simulink model "test_individual_beam_backup"  (R2013a)
settings: Solver=ode14x  StartTime=0.0  StopTime=3  FixedStep=1e-4  RelTol=1e-3
values from neighbouring files (symbols this model uses):
  A = [0 1 0 0 0 0;-2 0 2 0 0 0;0 0 0 1 0 0;2 0 -4 -3 2 3;0 0 0 0 0 1;0 0 2 3 -2 -3]    [AFSMC_Observer.m]    (also in AFSMC_Observer2.m = A(1:4,1:4); AFSMC_Observer2_with_alfa_beta.m = A(1:4,1:4); AFSMC_Observer2_with_alfa_beta_new.m = A(1:4,1:4); AFSMC_Observer_alfa_beta_new.m = A(1:4,1:4))
  B = [0 1 0 0 0 0;0 0 0 0 0 1]'    [AFSMC_Observer.m]    (also in AFSMC_Observer2.m = BB(1:4,1); AFSMC_Observer2_with_alfa_beta.m = BB(1:4,1); AFSMC_Observer2_with_alfa_beta_new.m = BB(1:4,1); AFSMC_Observer_alfa_beta_new.m = BB(1:4,1))
  C = rand(2,6)    [AFSMC_Observer.m]    (also in AFSMC_Observer2.m = C(1,1:4); AFSMC_Observer2_with_alfa_beta.m = C(1,1:4); AFSMC_Observer2_with_alfa_beta_new.m = C(1,1:4); AFSMC_Observer_alfa_beta_new.m = C(1,1:4))
  DeltaA = [0 0 0 0 0 0;2*ksi 0 -2*ksi 0 0 0;0 0 0 0 0 0;-2*ksi 0 4*ksi 3*ksi -2*ksi -3*ksi;0 0 0 0 0 1;0 0 -2*ksi -3*ksi 2*ksi 3*ksi]    [AFSMC_Observer.m]    (also in AFSMC_Observer2.m = A*0; AFSMC_Observer2_with_alfa_beta.m = A*0; AFSMC_Observer2_with_alfa_beta_new.m = A*0; AFSMC_Observer_alfa_beta_new.m = A*0)
  DeltaB = [0 -ksi 0 0 0 0;0 0 0 0 0 -ksi]'    [AFSMC_Observer.m]    (also in AFSMC_Observer2.m = B*0; AFSMC_Observer2_with_alfa_beta.m = B*0; AFSMC_Observer2_with_alfa_beta_new.m = B*0; AFSMC_Observer_alfa_beta_new.m = B*0)
  DeltaC = C*cm    [AFSMC_Observer.m]    (also in AFSMC_Observer2.m; AFSMC_Observer2_with_alfa_beta.m; AFSMC_Observer2_with_alfa_beta_new.m; AFSMC_Observer_alfa_beta_new.m)
  H = [0 1 0 0 0 0;0 0 0 1 0 0;0 0 0 0 0 1]'    [AFSMC_Observer.m]    (also in AFSMC_Observer2.m = BB(1:4,2); AFSMC_Observer2_with_alfa_beta.m = BB(1:4,2); AFSMC_Observer2_with_alfa_beta_new.m = BB(1:4,2); AFSMC_Observer_alfa_beta_new.m = BB(1:4,2))
  K = dec2mat(LMISYS3,xgen,4)    [AFSMC_Observer.m]    (also in AFSMC_Observer2.m = Kc; AFSMC_Observer2_with_alfa_beta.m = Kc; AFSMC_Observer_alfa_beta_new.m; AFSMC_Observer_backup2.m)
  L = dec2mat(LMISYS3,xgen,3)    [AFSMC_Observer.m]    (also in AFSMC_Observer2.m = Lo; AFSMC_Observer2_with_alfa_beta.m = Lo; AFSMC_Observer_alfa_beta_new.m; AFSMC_Observer_alfa_beta_withoutQ1Q2.m = dec2mat(LMISYS3,xgen,2))
settings Model: Creator=User  LastModifiedBy=User

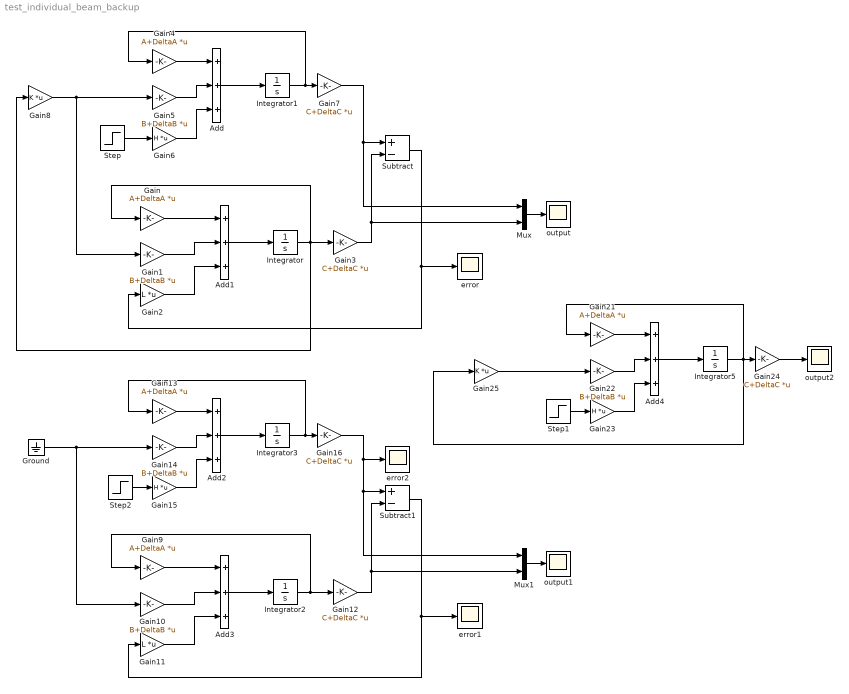
== system test_individual_beam_backup ==
  Add{,1..4} (5 alike) : Sum  Inputs=+++
  Gain{,4,9,13,21} (5 alike) : Gain  Gain=A+DeltaA  Multiplication=Matrix(K*u)
  Gain{1,5,10,14,22} (5 alike) : Gain  Gain=B+DeltaB  Multiplication=Matrix(K*u)
  Gain11 : Gain  Gain=L  Multiplication=Matrix(K*u)
  Gain{3,7,12,16,24} (5 alike) : Gain  Gain=C+DeltaC  Multiplication=Matrix(K*u)
  Gain15 : Gain  Gain=H  Multiplication=Matrix(K*u)
  Gain2 : Gain  Gain=L  Multiplication=Matrix(K*u)
  Gain23 : Gain  Gain=H  Multiplication=Matrix(K*u)
  Gain25 : Gain  Gain=K  Multiplication=Matrix(K*u)
  Gain6 : Gain  Gain=H  Multiplication=Matrix(K*u)
  Gain8 : Gain  Gain=K  Multiplication=Matrix(K*u)
  Ground : Ground
  Integrator{,1..3,5} (5 alike) : Integrator
  Mux : Mux  Inputs=2
  Mux1 : Mux  Inputs=2
  Step : Step  Time=0.001  Before=1  After=0  SampleTime=0
  Step1 : Step  Time=0.001  Before=1  After=0  SampleTime=0
  Step2 : Step  Time=0.001  Before=1  After=0  SampleTime=0
  Subtract : Sum  Inputs=+-
  Subtract1 : Sum  Inputs=+-
  error : Scope
      settings: SaveName=ScopeData2
  error1 : Scope
  error2 : Scope
      settings: SaveName=ScopeData4
  output : Scope
  output1 : Scope
      settings: SaveName=ScopeData3
  output2 : Scope
      settings: SaveName=ScopeData5
  wires:
  Add1/1 -> Integrator/1
  Gain/1 -> Add1/1
  Gain1/1 -> Add1/2
  Gain2/1 -> Add1/3
  Add/1 -> Integrator1/1
  Integrator1/1 -> Gain7/1, Gain4/1
  Gain4/1 -> Add/1
  Gain5/1 -> Add/2
  Gain8/1 -> Gain1/1, Gain5/1
  Gain6/1 -> Add/3
  Mux/1 -> output/1
  Gain7/1 -> Mux/1, Subtract/1
  Gain3/1 -> Subtract/2, Mux/2
  Subtract/1 -> error/1, Gain2/1
  Integrator/1 -> Gain8/1, Gain3/1, Gain/1
  Add3/1 -> Integrator2/1
  Gain9/1 -> Add3/1
  Gain10/1 -> Add3/2
  Gain11/1 -> Add3/3
  Add2/1 -> Integrator3/1
  Integrator3/1 -> Gain16/1, Gain13/1
  Gain13/1 -> Add2/1
  Gain14/1 -> Add2/2
  Ground/1 -> Gain10/1, Gain14/1
  Gain15/1 -> Add2/3
  Mux1/1 -> output1/1
  Gain16/1 -> error2/1, Mux1/1, Subtract1/1
  Gain12/1 -> Subtract1/2, Mux1/2
  Subtract1/1 -> error1/1, Gain11/1
  Integrator2/1 -> Gain12/1, Gain9/1
  Add4/1 -> Integrator5/1
  Gain21/1 -> Add4/1
  Gain22/1 -> Add4/2
  Gain25/1 -> Gain22/1
  Gain23/1 -> Add4/3
  Step1/1 -> Gain23/1
  Gain24/1 -> output2/1
  Integrator5/1 -> Gain25/1, Gain21/1, Gain24/1
  Step/1 -> Gain6/1
  Step2/1 -> Gain15/1
